simulink model "DMS_TEST"  (Simulink 8.1)
settings: Solver=ode4  StartTime=0.0  StopTime=inf  FixedStep=Ts  MaxStep=1e-3  RelTol=1e-3
model workspace (MAT data in the model file):
  op_snapshot1 : opcond.OperatingPoint (value not decoded)
PostLoadFcn:
  | INTEGRATION_TEST_01_init;
InitFcn:
  | INTEGRATION_TEST_01_init;
values from neighbouring files (symbols this model uses):
  Ts = 100E-6    (= 0.0001)    [INTEGRATION_TEST_01_init.m]
undefined symbols (not defined in the file or in its folder): CMD_signals
libraries: artemis x1, rtio_generic_modbus x1, powerlib x1
settings Model: ARTEMISmethode_block_infos=$$__separator__$$DMS_TEST/ARTEMIS Guide$$__separator__$$  Creator=RE25624  LastModifiedBy=re25624  BufferReuse=off
settings SolverCC: ZeroCrossAlgorithm=Adaptive
settings DataIOCC: ExternalInput=getinputstruct(op_snapshot1)  InitialState=getstatestruct(op_snapshot1)  LimitDataPoints=off  MaxDataPoints=90060  SignalLoggingSaveFormat=Dataset  SaveOutput=off  SignalLogging=off  DSMLogging=off  SaveTime=off  OutputSaveName=result
settings OptimizationCC: BlockReduction=off  OptimizeBlockIOStorage=off  BufferReuse=off  ExpressionFolding=off  LocalBlockOutputs=off
settings DebuggingCC: MaxConsecutiveZCsMsg=warning  IgnoredZcDiagnostic=none  SolverPrmCheckMsg=none  MultiTaskRateTransMsg=warning  FcnCallInpInsideContextMsg=EnableAllAsWarning  FrameProcessingCompatibilityMsg=error  ModelReferenceExtraNoncontSigs=warning  StrictBusMsg=None
settings ModelReferenceCC: UpdateModelReferenceTargets=IfOutOfDate
settings SFSimCC: SFSimEcho=off
settings GRTTargetCC: CodeReplacementLibrary=C89/C90 (ANSI)

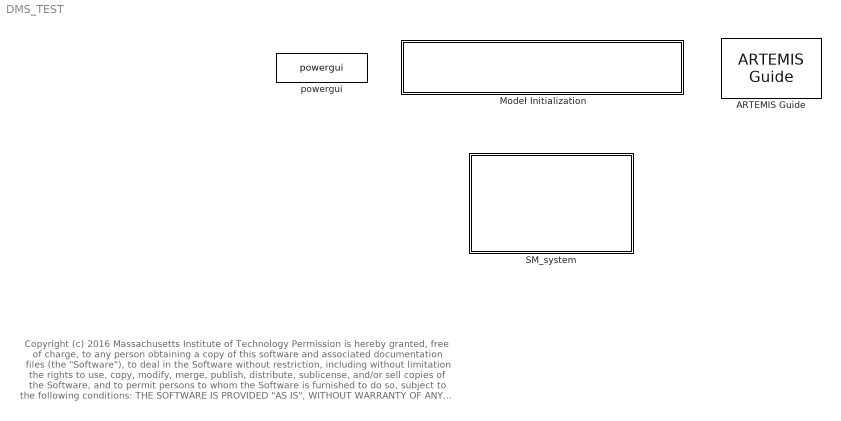
== system DMS_TEST ==
  note: Copyright (c) 2016 Massachusetts Institute of Technology
      | Permission is hereby granted, free of charge, to any person obtaining a copy of this software and associated documentation files (the "Software"), to deal
      | in the Software without restriction, including without limitation the rights to use, copy, modify, merge, publish, distribute, sublicense, and/or sell copies of the
      | Software, and to permit persons to whom the Software is furnished to do so, subject to the following conditions:
      |
      | THE SOFTWARE IS PROVIDED "AS IS", WITHOUT WARRANTY OF ANY KIND, EXPRESS OR IMPLIED, INCLUDING BUT NOT LIMITED TO THE
      | WARRANTIES OF MERCHANTABILITY, FITNESS FOR A PARTICULAR PURPOSE AND NONINFRINGEMENT. IN NO EVENT SHALL THE AUTHORS
      | OR COPYRIGHT HOLDERS BE LIABLE FOR ANY CLAIM, DAMAGES OR OTHER LIABILITY, WHETHER IN AN ACTION OF CONTRACT, TORT OR
      | OTHERWISE, ARISING FROM, OUT OF OR IN CONNECTION WITH THE SOFTWARE OR THE USE OR OTHER DEALINGS IN THE SOFTWARE.
  ARTEMIS Guide : artemis/ARTEMIS/ARTEMIS Guide  Tag=FTSSmethode_opal_4hx0r99  Description=5.0_z1  lock=on  Ts=Ts  opt=art5  dyna=off  nb_perm=4  RT_fullcomp=off  ssn=on  ssn_itvc=off  ssn_ivic=off  ssn_ext=off  ssn_solver=Art5 with Backward Euler nodal interface  ssn_impulse=off  ssn_quasimpulse=off  ssn_impulse_loop=2  paraExtinctionThy=off  Thy_Impulse=on  dtc=Off  dtc_opt=normal  ao=on  simtype=off  ct_mac=off  lin_mov=off  lsp=[0.001 2]  spike_skip=Disabled  dtc_extra=1  dtc_sws=normal  dtc_pied=0.5  SPSRulesBlock=SPSRules  tre=on  ctmm=off  LF=off  dpl_type=ARTEMiS DPL  rlc_type=off  custom_type=off  para=on  ssn_ImpulseLoopBlockedStateUpdate=2  ssn_mov_iter_number=5  ssn_switch_iter_number=5
  Model Initialization : Subsystem  AncestorBlock=artemis/Tools /Misc/Model Initialization  mask(Model Functions){InitFcnX=INTEGRATION_TEST_01_init;, prel=off, posl=on, inif=on, strf=off}
      mask prompts: InitFcnX "Initialisation"; prel "Preload Function"; posl "PostLoad Function"; inif "InitFcn"; strf "StartFcn"
      mask init:
      | currentBlock = gcb;
      | root = bdroot(currentBlock);
      | 
      | 
      | if ~strcmp(get_param(root,'BlockDiagramType'),'library')
      |     if prel==1
      |         set_param(root, 'PreLoadFcn', InitFcnX);
      |     else
      |         set_param(root, 'PreLoadFcn', '');
      |     end
      |     if inif==1
      |         set_param(root, 'InitFcn', InitFcnX);
      |     else
      |         set_param(root, 'InitFcn', '');
      |     end
      |     if strf==1
      |         set_param(root, 'StartFcn', InitFcnX);
      |     else
      |         set_param(root, 'StartFcn', '');
      |     end
      |     if posl==1
      |         set_param(root, 'PostLoadFcn', InitFcnX);
      |     else
      |         set_param(root, 'PostLoadFcn', '');
      |     end
      | end
      | 
      | pos = get_param(currentBlock, 'Position');
      | width = pos(3) - pos(1); height = pos(4) - pos(2);
      | txt = [ upper(root) '\n' '- InitFcn. . . . . '  get_param(root, 'InitFcn') ];
      settings: CopyFcn=set_param(gcb,'LinkStatus','inactive')
      mask Display: text(5, height*0.5, txt, 'horizontalAlignment', 'left', 'verticalAlignment', 'middle') ;
  SM_system : Subsystem
  powergui : powerlib/powergui  Priority=2  SimulationMode=Discrete  SolverType=Tustin  SampleTime=Ts  frequency=60  SPID=off  DisableSnubberDevices=off  DisableRonSwitches=off  DisableVfSwitches=off  SwTol=0  Interpol=off  DisplayEquations=off  frequencyindice=0  Pbase=100e6  ErrMax=1e-4  Iterations=50  UnitsV=kV  UnitsW=MW  FunctionMessages=off  echomessages=off  HookPort=off  EnableUseOfTLC=off  x0status=blocks  RestoreLinks=warning  ResistiveCurrentMeasurement=off  Frange=logspace(0,3,50)  Ylog=off  Xlog=off  ShowGrid=off  save=off  variable=ZData  structure=0  ZoomFFT=on  StartTime=0.0  cycles=2  DisplayStyle=off  fundamental=60  FreqAxis=off  MaxFrequency=1000  frequencyindicesteady=1  RmsSteady=1  display=off  Ts=0  methode=off

== system DMS_TEST/Model Initialization ==

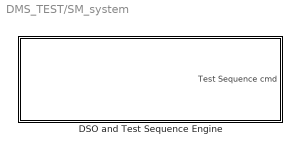
== system DMS_TEST/SM_system ==
  DSO and Test Sequence Engine : Subsystem

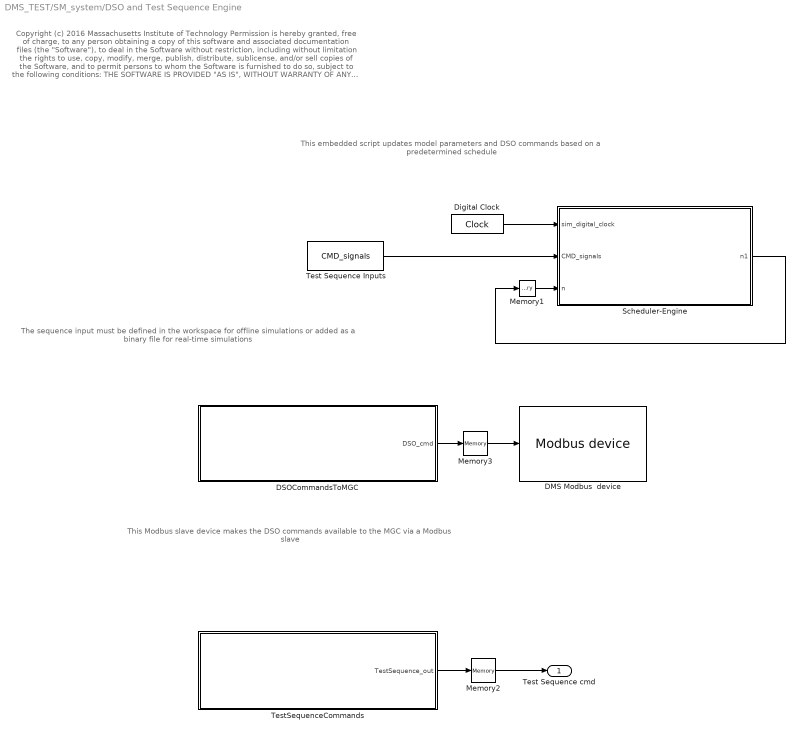
== system DMS_TEST/SM_system/DSO and Test Sequence Engine ==
  note: This Modbus slave device makes the DSO
      | commands available to the MGC via a Modbus slave
  note: This embedded script updates model  parameters
      | and DSO commands based on a predetermined schedule
  note: Copyright (c) 2016 Massachusetts Institute of Technology
      | Permission is hereby granted, free of charge, to any person obtaining a copy of this software and associated documentation files (the "Software"), to deal
      | in the Software without restriction, including without limitation the rights to use, copy, modify, merge, publish, distribute, sublicense, and/or sell copies of the
      | Software, and to permit persons to whom the Software is furnished to do so, subject to the following conditions:
      |
      | THE SOFTWARE IS PROVIDED "AS IS", WITHOUT WARRANTY OF ANY KIND, EXPRESS OR IMPLIED, INCLUDING BUT NOT LIMITED TO THE
      | WARRANTIES OF MERCHANTABILITY, FITNESS FOR A PARTICULAR PURPOSE AND NONINFRINGEMENT. IN NO EVENT SHALL THE AUTHORS
      | OR COPYRIGHT HOLDERS BE LIABLE FOR ANY CLAIM, DAMAGES OR OTHER LIABILITY, WHETHER IN AN ACTION OF CONTRACT, TORT OR
      | OTHERWISE, ARISING FROM, OUT OF OR IN CONNECTION WITH THE SOFTWARE OR THE USE OR OTHER DEALINGS IN THE SOFTWARE.
  note: The sequence input must be defined in the
      | workspace for offline simulations
      |
      | or added as a binary file for real-time simulations
  DMS Modbus  device : rtio_generic_modbus/Modbus device  conf_name=DMS_slave_cfg.opal  conf_name_mask=DMS_slave_cfg.xls  sample_time=0
  DSOCommandsToMGC : Subsystem  mask(DSOCommandsToMGC){DSO_Start_Time=0, DSO_Duration=0, DSO_Disconnect=0, DSO_Export=0, Import_Export_Value=0, DSO_PF_Support=0, PF_Value=0, DSO_VAR_Support=0, VAR_Value=0}
      mask prompts: DSO_Start_Time "DSO start time"; DSO_Duration "DSO duration"; DSO_Disconnect "DSO disconnect"; DSO_Export "DSO kW export (1) or Import limits (0)"; Import_Export_Value "Export/Import value [kW]"; DSO_PF_Support "DSO PF support (1) or Not (0)"; PF_Value "System PF value [+(lag) or -(lead)]"; DSO_VAR_Support "DSO VAR support (1) or Not (0)"; VAR_Value "Import/Export value [kVAr]"
      mask help:
      | This block sends Distribution System Operator (DSO) commands over Modbus to the microgrid controller (MGC) to define the microgrid interaction with the grid. All commands are synchronized to the start-time and duration-time, and are viewed as from the grid side.
      |
      | - List of requests in order sent to Modbus
      |
      | DSO start time: start time for the MGC to execute the given command
      |
      | DSO duration: duration time of given command
      |
      | DSO disconnect: microgrid disconnect request
      |
      | DSO kW export (1) or Import limits (0): request for real power export/import limits
      |
      | Export/Import value [kW]: defined real power export/import value
      |
      | DSO PF support (1) or Not (0): power factor support request
      |
      | System PF value [+(lag) or -(lead)]: requested system power factor
      |
      | DSO VAR support (1) or Not (0): request for reactive power support
      |
      | Export value [kVAr]: defined reactive power export value
  Digital Clock : DigitalClock  SampleTime=Ts
  Memory1 : Memory  X0=1
  Memory2 : Memory
  Memory3 : Memory
  Scheduler-Engine : MATLAB Function  TreatAsAtomicUnit=on
  Test Sequence Inputs : Constant  Value=CMD_signals
  TestSequenceCommands : Subsystem  mask(TestSequenceCommands){fault1=0, fault2=0, fault3=0, fault4=0, fault5=0, fault6=0, fault7=0, fault8=0, load_gain=0.75}
      mask prompts: fault1 "Fault 1"; fault2 "Fault 2"; fault3 "Fault 3"; fault4 "Fault 4"; fault5 "Fault 5"; fault6 "Fault 6"; fault7 "Fault 7"; fault8 "Fault 8"; load_gain "System Load Gain"
      mask help:
      | Real-Time: Block is automatically updated during the simulation
      | Off-line: User needs to apply faults or vary loads manually
      |
      | Fault #1..8: Booleans used to activate faults in the system - currently, up to 8 locations for Banshee.
      | Load gain: Factors to vary the overall system load.
  Test Sequence cmd : Outport
  wires:
  Scheduler-Engine/1(n1) -> Memory1/1
  Memory1/1 -> Scheduler-Engine/3(n)
  Test Sequence Inputs/1 -> Scheduler-Engine/2(CMD_signals)
  Digital Clock/1 -> Scheduler-Engine/1(sim_digital_clock)
  DSOCommandsToMGC/1(DSO_cmd) -> Memory3/1
  TestSequenceCommands/1(TestSequence_out) -> Memory2/1
  Memory2/1 -> Test Sequence cmd/1
  Memory3/1 -> DMS Modbus  device/1

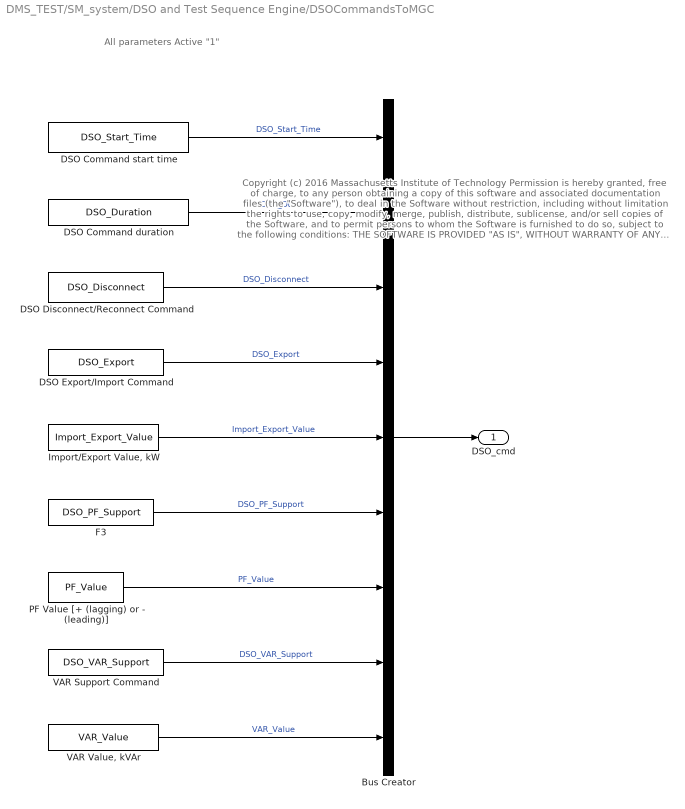
== system DMS_TEST/SM_system/DSO and Test Sequence Engine/DSOCommandsToMGC ==
  note: All parameters Active "1"
  note: Copyright (c) 2016 Massachusetts Institute of Technology
      | Permission is hereby granted, free of charge, to any person obtaining a copy of this software and associated documentation files (the "Software"), to deal
      | in the Software without restriction, including without limitation the rights to use, copy, modify, merge, publish, distribute, sublicense, and/or sell copies of the
      | Software, and to permit persons to whom the Software is furnished to do so, subject to the following conditions:
      |
      | THE SOFTWARE IS PROVIDED "AS IS", WITHOUT WARRANTY OF ANY KIND, EXPRESS OR IMPLIED, INCLUDING BUT NOT LIMITED TO THE
      | WARRANTIES OF MERCHANTABILITY, FITNESS FOR A PARTICULAR PURPOSE AND NONINFRINGEMENT. IN NO EVENT SHALL THE AUTHORS
      | OR COPYRIGHT HOLDERS BE LIABLE FOR ANY CLAIM, DAMAGES OR OTHER LIABILITY, WHETHER IN AN ACTION OF CONTRACT, TORT OR
      | OTHERWISE, ARISING FROM, OUT OF OR IN CONNECTION WITH THE SOFTWARE OR THE USE OR OTHER DEALINGS IN THE SOFTWARE.
  Bus Creator : BusCreator  Inputs=9
  DSO Command duration : Constant  Value=DSO_Duration
  DSO Command start time : Constant  Value=DSO_Start_Time
  DSO Disconnect/Reconnect Command : Constant  Value=DSO_Disconnect
  DSO Export/Import Command : Constant  Value=DSO_Export
  F3 : Constant  Value=DSO_PF_Support
  "Import/Export Value, kW" : Constant  Value=Import_Export_Value
  PF Value [+ (lagging) or - (leading)] : Constant  Value=PF_Value
  VAR Support Command : Constant  Value=DSO_VAR_Support
  "VAR Value, kVAr" : Constant  Value=VAR_Value
  DSO_cmd : Outport
  wires:
  "Import/Export Value, kW"/1 -> Bus Creator/5  "Import_Export_Value"
  DSO Command duration/1 -> Bus Creator/2  "DSO_Duration"
  DSO Command start time/1 -> Bus Creator/1  "DSO_Start_Time"
  PF Value [+ (lagging) or - (leading)]/1 -> Bus Creator/7  "PF_Value"
  "VAR Value, kVAr"/1 -> Bus Creator/9  "VAR_Value"
  VAR Support Command/1 -> Bus Creator/8  "DSO_VAR_Support"
  F3/1 -> Bus Creator/6  "DSO_PF_Support"
  DSO Export/Import Command/1 -> Bus Creator/4  "DSO_Export"
  DSO Disconnect/Reconnect Command/1 -> Bus Creator/3  "DSO_Disconnect"
  Bus Creator/1 -> DSO_cmd/1

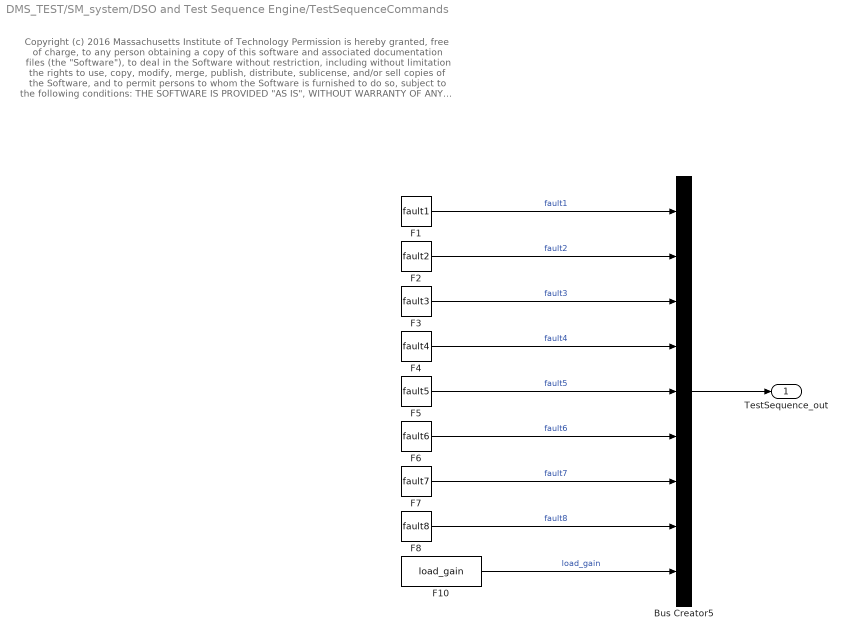
== system DMS_TEST/SM_system/DSO and Test Sequence Engine/TestSequenceCommands ==
  note: Copyright (c) 2016 Massachusetts Institute of Technology
      | Permission is hereby granted, free of charge, to any person obtaining a copy of this software and associated documentation files (the "Software"), to deal
      | in the Software without restriction, including without limitation the rights to use, copy, modify, merge, publish, distribute, sublicense, and/or sell copies of the
      | Software, and to permit persons to whom the Software is furnished to do so, subject to the following conditions:
      |
      | THE SOFTWARE IS PROVIDED "AS IS", WITHOUT WARRANTY OF ANY KIND, EXPRESS OR IMPLIED, INCLUDING BUT NOT LIMITED TO THE
      | WARRANTIES OF MERCHANTABILITY, FITNESS FOR A PARTICULAR PURPOSE AND NONINFRINGEMENT. IN NO EVENT SHALL THE AUTHORS
      | OR COPYRIGHT HOLDERS BE LIABLE FOR ANY CLAIM, DAMAGES OR OTHER LIABILITY, WHETHER IN AN ACTION OF CONTRACT, TORT OR
      | OTHERWISE, ARISING FROM, OUT OF OR IN CONNECTION WITH THE SOFTWARE OR THE USE OR OTHER DEALINGS IN THE SOFTWARE.
  Bus Creator5 : BusCreator  Inputs=9
  F1 : Constant  Value=fault1
  F10 : Constant  Value=load_gain
  F2 : Constant  Value=fault2
  F3 : Constant  Value=fault3
  F4 : Constant  Value=fault4
  F5 : Constant  Value=fault5
  F6 : Constant  Value=fault6
  F7 : Constant  Value=fault7
  F8 : Constant  Value=fault8
  TestSequence_out : Outport
  wires:
  F1/1 -> Bus Creator5/1  "fault1"
  F2/1 -> Bus Creator5/2  "fault2"
  F3/1 -> Bus Creator5/3  "fault3"
  F4/1 -> Bus Creator5/4  "fault4"
  F6/1 -> Bus Creator5/6  "fault6"
  F7/1 -> Bus Creator5/7  "fault7"
  F5/1 -> Bus Creator5/5  "fault5"
  F8/1 -> Bus Creator5/8  "fault8"
  F10/1 -> Bus Creator5/9  "load_gain"
  Bus Creator5/1 -> TestSequence_out/1

== matlab function SM_system/DSO and Test Sequence Engine/Scheduler-Engine ==
  data: sim_digital_clock input double; CMD_signals input double; n input double; n1 output double
% Copyright (c) 2016 Massachusetts Institute of Technology
% Permission is hereby granted, free of charge, to any person obtaining a copy of this software and associated documentation files (the "Software"), to deal
% in the Software without restriction, including without limitation the rights to use, copy, modify, merge, publish, distribute, sublicense, and/or sell copies of the
% Software, and to permit persons to whom the Software is furnished to do so, subject to the following conditions:
%
% THE SOFTWARE IS PROVIDED "AS IS", WITHOUT WARRANTY OF ANY KIND, EXPRESS OR IMPLIED, INCLUDING BUT NOT LIMITED TO THE
% WARRANTIES OF MERCHANTABILITY, FITNESS FOR A PARTICULAR PURPOSE AND NONINFRINGEMENT. IN NO EVENT SHALL THE AUTHORS
% OR COPYRIGHT HOLDERS BE LIABLE FOR ANY CLAIM, DAMAGES OR OTHER LIABILITY, WHETHER IN AN ACTION OF CONTRACT, TORT OR
% OTHERWISE, ARISING FROM, OUT OF OR IN CONNECTION WITH THE SOFTWARE OR THE USE OR OTHER DEALINGS IN THE SOFTWARE.
%


function n1  = scheduler_engine(sim_digital_clock,CMD_signals,n)

% This function takes in the test sequence signals (vector) from a *.mat file
% externally generated with TestProcedure_xlsRead.m. The function updates parameters
% within the simulink model for DMS and TST (test sequence) according a given time stamp

% **** Sequence signal vector order ****
% CMD column 1 = time
% CMD column 2 = POI feeder 1 SEL relay
% CMD column 3 = POI feeder 2 SEL relay
% CMD column 4 = POI feeder 3 SEL relay
% CMD column 5 = diesel breaker
% CMD column 6 = solar irradiance gain
% CMD column 7 = solar breaker
% CMD column 8 = CHP breaker
% CMD column 9 = load gain
% CMD column 10 = motor 1 breaker
% CMD column 11 = motor 2 breaker
% CMD column 12 = fault location 1
% CMD column 13 = fault location 2
% CMD column 14 = fault location 3
% CMD column 15 = fault location 4
% CMD column 16 = fault location 5
% CMD column 17 = fault location 6
% CMD column 18 = fault location 7
% CMD column 19 = fault location 8 SECT
%
% Next section is for dso modbus slave
%
% CMD column 20 = dso Disconnect command
% CMD column 21 = dso Reconnect command
% CMD column 22 = dso Export command
% CMD column 23 = dso Import command
% CMD column 24 = dso power factor command
% CMD column 25 = dso VAR support command
% CMD column 26 = dso Demand Response command
% CMD column 27 = dso Import/export value
% CMD column 28 = dso power factor value
% CMD column 29 = dso VAR value
% CMD column 30 = dso DR value
% CMD column 31 = dso Command start time
% CMD column 32 = dso command duration


coder.extrinsic('set_param') %declare set_param as an extrinsic function
coder.extrinsic('num2str') %declare num2str as an extrinsic function

time = CMD_signals(:,1);
% time_lastCMD = time(length(time)); %do i need this anymore?
numCMDs = length(time);

% indicate where in the simulink model is the test sequence block located
TST_SEQ_block_location = 'DMS_TEST/SM_system/DSO and Test Sequence Engine/';

if n > numCMDs   % do nothing if we have exhausted all commands
    n1 = n;
else
    if sim_digital_clock > time(n) % when the simulation time is greater than the command signal time, execute set_param
        n1 = n+1; % increment to next command to execute
        
        % parameters to set within simulink model
        set_param([TST_SEQ_block_location, 'TestSequenceCommands'],...
            'load_gain', num2str(CMD_signals(n,9)),...
            'fault1',    num2str(CMD_signals(n,12)),...
            'fault2',    num2str(CMD_signals(n,13)),...
            'fault3',    num2str(CMD_signals(n,14)),...
            'fault4',    num2str(CMD_signals(n,15)),...
            'fault5',    num2str(CMD_signals(n,16)),...
            'fault6',    num2str(CMD_signals(n,17)),...
            'fault7',    num2str(CMD_signals(n,18)),...
            'fault8',    num2str(CMD_signals(n,19)));
        %%%
        set_param([TST_SEQ_block_location, 'DSOCommandsToMGC'],...
            'DSO_Start_Time',      num2str(CMD_signals(n,31)),...
            'DSO_Duration',        num2str(CMD_signals(n,32)),...
            'DSO_Disconnect',      num2str(CMD_signals(n,20)),...
            'DSO_Export',          num2str(CMD_signals(n,22)),...
            'Import_Export_Value', num2str(CMD_signals(n,27)),...
            'DSO_PF_Support',      num2str(CMD_signals(n,24)),...
            'PF_Value',            num2str(CMD_signals(n,28)),...
            'DSO_VAR_Support',     num2str(CMD_signals(n,25)),...
            'VAR_Value',           num2str(CMD_signals(n,30)));
        
    else  % wait until the simulation time has eclisped the next command time
        n1 = n;
    end
end
